simulink model "Architecture"  (R2025b)
settings: configuration reference "simulation" (kept outside this file)
StopFcn:
  | sim("models\PlaybackMechExplorer");
settings Model: DataDictionary=test.sldd  Creator=rpumpo  LastModifiedBy=rpumpo
settings ConfigSetRef: SourceName=simulation

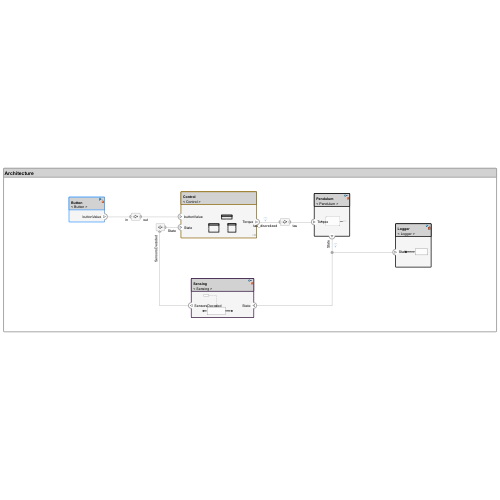
[thumbnail: Simulink's stored preview of the top-level diagram]
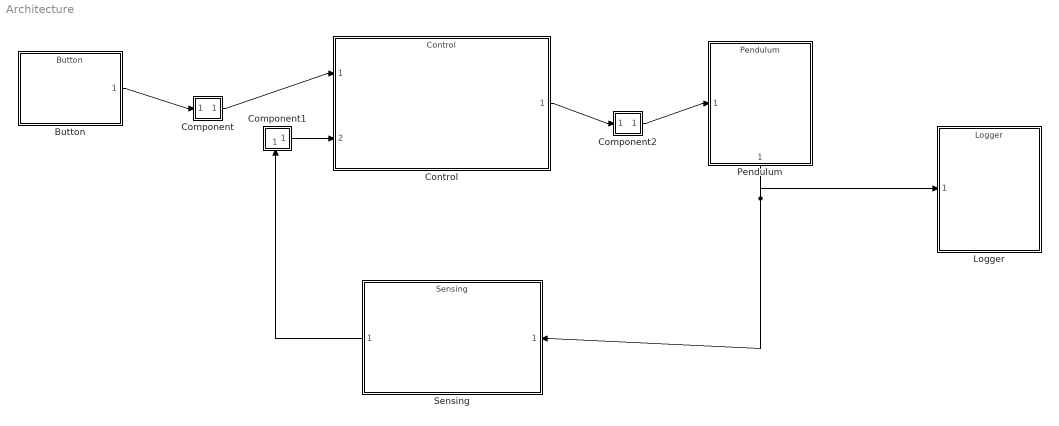
== system Architecture ==
  Button : ModelReference  ModelNameDialog=Button  SimulationMode=Normal  ModelReferenceVersion=1.6
      settings: PortSchema="{\"entries\":[{\"content\":{\"headerSize\":38,\"margin\":15,\"minimumSpacing\":25,\"sides\":[{\"content\":{},\"type\":\"ConnectorPlacement.EquallySpacedRectSide\",\"uuid\":\"8ec1d587-685a-426d-afd8-122ee0061f4c\"},{\"content\":{\"connectorIds\":[\"Out1\"],\"side\":\"RIGHT\"},\"type\":\"ConnectorPlacement.EquallySpacedRectSide\",\"uuid\":\"676e5b40-739e-4f92-aeaf-bee5408ade44\"},{\"content\":{\"side\":\"TOP\"},\"type\":\"ConnectorPlacement.EquallySpacedRectSide\",\"uuid\":\"01bc015e-a21d-4ad7-afeb-e19c798ece57\"}]},\"type\":\"ConnectorPlacement.EquallySpacedConnector\",\"uuid\":\"c5b56a8a-bb96-4a1a-b5ae-768463cc4daa\"}],\"packageUris\":[\"http://schema.mathworks.com/mf0/Connector/R2020b\"],\"version\":\"1.0\"}"
  Component : Subsystem
      settings: PortSchema="{\"entries\":[{\"content\":{\"margin\":10,\"minimumSpacing\":15,\"sides\":[{\"content\":{\"connectorIds\":[\"In1\"]},\"type\":\"ConnectorPlacement.EquallySpacedRectSide\",\"uuid\":\"52fbcab2-77e6-4c43-8240-cdc79aed3b18\"},{\"content\":{\"connectorIds\":[\"Out1\"],\"side\":\"RIGHT\"},\"type\":\"ConnectorPlacement.EquallySpacedRectSide\",\"uuid\":\"cdca0b56-8fb5-4ee8-9ac9-94cbfddd1752\"},{\"content\":{\"side\":\"TOP\"},\"type\":\"ConnectorPlacement.EquallySpacedRectSide\",\"uuid\":\"eb715b44-d91d-4d1d-af0d-8b01d7a8babe\"}]},\"type\":\"ConnectorPlacement.EquallySpacedConnector\",\"uuid\":\"fecc88ef-e61f-4ca4-bc17-41110eeb9f29\"}],\"packageUris\":[\"http://schema.mathworks.com/mf0/Connector/R2020b\"],\"version\":\"1.0\"}"
  Component1 : Subsystem
      settings: PortSchema="{\"entries\":[{\"content\":{\"margin\":10,\"minimumSpacing\":15,\"sides\":[{\"content\":{},\"type\":\"ConnectorPlacement.EquallySpacedRectSide\",\"uuid\":\"52fbcab2-77e6-4c43-8240-cdc79aed3b18\"},{\"content\":{\"connectorIds\":[\"Out1\"],\"side\":\"RIGHT\"},\"type\":\"ConnectorPlacement.EquallySpacedRectSide\",\"uuid\":\"cdca0b56-8fb5-4ee8-9ac9-94cbfddd1752\"},{\"content\":{\"side\":\"TOP\"},\"type\":\"ConnectorPlacement.EquallySpacedRectSide\",\"uuid\":\"eb715b44-d91d-4d1d-af0d-8b01d7a8babe\"},{\"content\":{\"connectorIds\":[\"In1\"],\"side\":\"BOTTOM\"},\"type\":\"ConnectorPlacement.EquallySpacedRectSide\",\"uuid\":\"c2091c5b-8a67-42b6-aad5-651c68393b83\"}]},\"type\":\"ConnectorPlacement.EquallySpacedConnector\",\"uuid\":\"fecc88ef-e61f-4ca4-bc17-41110eeb9f29\"}],\"packageUris\":[\"http://schema.mathworks.com/mf0/Connector/R2020b\"],\"version\":\"1.0\"}"
  Component2 : Subsystem
      settings: PortSchema="{\"entries\":[{\"content\":{\"margin\":10,\"minimumSpacing\":15,\"sides\":[{\"content\":{\"connectorIds\":[\"In1\"]},\"type\":\"ConnectorPlacement.EquallySpacedRectSide\",\"uuid\":\"52fbcab2-77e6-4c43-8240-cdc79aed3b18\"},{\"content\":{\"connectorIds\":[\"Out1\"],\"side\":\"RIGHT\"},\"type\":\"ConnectorPlacement.EquallySpacedRectSide\",\"uuid\":\"cdca0b56-8fb5-4ee8-9ac9-94cbfddd1752\"},{\"content\":{\"side\":\"TOP\"},\"type\":\"ConnectorPlacement.EquallySpacedRectSide\",\"uuid\":\"eb715b44-d91d-4d1d-af0d-8b01d7a8babe\"}]},\"type\":\"ConnectorPlacement.EquallySpacedConnector\",\"uuid\":\"fecc88ef-e61f-4ca4-bc17-41110eeb9f29\"}],\"packageUris\":[\"http://schema.mathworks.com/mf0/Connector/R2020b\"],\"version\":\"1.0\"}"
  Control : ModelReference  ModelNameDialog=Control  SimulationMode=Normal  ScheduleRates=on  ModelReferenceVersion=1.56
      settings: PortSchema="{\"entries\":[{\"content\":{\"headerSize\":38,\"margin\":15,\"minimumSpacing\":25,\"sides\":[{\"content\":{\"connectorIds\":[\"In1\",\"In2\"]},\"type\":\"ConnectorPlacement.EquallySpacedRectSide\",\"uuid\":\"863a0b16-e36b-44d6-9477-1468a80c696d\"},{\"content\":{\"connectorIds\":[\"Out1\"],\"side\":\"RIGHT\"},\"type\":\"ConnectorPlacement.EquallySpacedRectSide\",\"uuid\":\"ac9067ee-3fe6-46b1-b4d3-b466d54413ae\"},{\"content\":{\"side\":\"TOP\"},\"type\":\"ConnectorPlacement.EquallySpacedRectSide\",\"uuid\":\"d4aa2d7a-4362-47d2-9788-fc41168b683c\"}]},\"type\":\"ConnectorPlacement.EquallySpacedConnector\",\"uuid\":\"884a1123-87f2-4a92-8ca9-5d4169531818\"}],\"packageUris\":[\"http://schema.mathworks.com/mf0/Connector/R2020b\"],\"version\":\"1.0\"}"
  Logger : ModelReference  ModelNameDialog=Logger.slx  SimulationMode=Normal  ModelReferenceVersion=1.9
      settings: PortSchema="{\"entries\":[{\"content\":{\"headerSize\":38,\"margin\":15,\"minimumSpacing\":25,\"sides\":[{\"content\":{\"connectorIds\":[\"In1\"]},\"type\":\"ConnectorPlacement.EquallySpacedRectSide\",\"uuid\":\"e3850213-7836-4a76-9138-db9561f2dfa3\"},{\"content\":{\"side\":\"RIGHT\"},\"type\":\"ConnectorPlacement.EquallySpacedRectSide\",\"uuid\":\"0376d83e-b2c6-47e1-ac72-ef48c291ef7a\"},{\"content\":{\"side\":\"TOP\"},\"type\":\"ConnectorPlacement.EquallySpacedRectSide\",\"uuid\":\"0ca152af-581b-44cc-8c1a-1940fec58944\"},{\"content\":{\"side\":\"BOTTOM\"},\"type\":\"ConnectorPlacement.EquallySpacedRectSide\",\"uuid\":\"58a901f2-a9fb-4ea5-a869-3facdef2b65b\"}]},\"type\":\"ConnectorPlacement.EquallySpacedConnector\",\"uuid\":\"7f3a45e2-30ac-43d0-98f3-5299d75cc4ed\"}],\"packageUris\":[\"http://schema.mathworks.com/mf0/Connector/R2020b\"],\"version\":\"1.0\"}"
  Pendulum : ModelReference  ModelNameDialog=Pendulum  SimulationMode=Normal  ModelReferenceVersion=1.26
      settings: PortSchema="{\"entries\":[{\"content\":{\"headerSize\":38,\"margin\":15,\"minimumSpacing\":25,\"sides\":[{\"content\":{\"connectorIds\":[\"In1\"]},\"type\":\"ConnectorPlacement.EquallySpacedRectSide\",\"uuid\":\"de57860b-0736-4135-a3e8-86dccc8271d5\"},{\"content\":{\"side\":\"RIGHT\"},\"type\":\"ConnectorPlacement.EquallySpacedRectSide\",\"uuid\":\"36ab646b-84bc-41af-8fac-a30bd324c6d3\"},{\"content\":{\"side\":\"TOP\"},\"type\":\"ConnectorPlacement.EquallySpacedRectSide\",\"uuid\":\"400916d0-a027-46ef-830f-ede2528573e4\"},{\"content\":{\"connectorIds\":[\"Out1\"],\"side\":\"BOTTOM\"},\"type\":\"ConnectorPlacement.EquallySpacedRectSide\",\"uuid\":\"00a68dd3-bf65-408f-b5a8-975bdf578244\"}]},\"type\":\"ConnectorPlacement.EquallySpacedConnector\",\"uuid\":\"8bf5b967-d017-4010-a731-66d331b6151a\"}],\"packageUris\":[\"http://schema.mathworks.com/mf0/Connector/R2020b\"],\"version\":\"1.0\"}"
  Sensing : ModelReference  ModelNameDialog=Sensing  SimulationMode=Normal  ScheduleRates=on  CachedPortDiscreteRates=[-1]  ModelReferenceVersion=1.10
      settings: PortSchema="{\"entries\":[{\"content\":{\"headerSize\":38,\"margin\":15,\"minimumSpacing\":25,\"sides\":[{\"content\":{\"connectorIds\":[\"Out1\"]},\"type\":\"ConnectorPlacement.EquallySpacedRectSide\",\"uuid\":\"863a0b16-e36b-44d6-9477-1468a80c696d\"},{\"content\":{\"connectorIds\":[\"In1\"],\"side\":\"RIGHT\"},\"type\":\"ConnectorPlacement.EquallySpacedRectSide\",\"uuid\":\"ac9067ee-3fe6-46b1-b4d3-b466d54413ae\"},{\"content\":{\"side\":\"TOP\"},\"type\":\"ConnectorPlacement.EquallySpacedRectSide\",\"uuid\":\"d4aa2d7a-4362-47d2-9788-fc41168b683c\"},{\"content\":{\"side\":\"HIDDEN\"},\"type\":\"ConnectorPlacement.EquallySpacedRectSide\",\"uuid\":\"a4bb201e-c22d-4356-a85f-9b291461f392\"}]},\"type\":\"ConnectorPlacement.EquallySpacedConnector\",\"uuid\":\"884a1123-87f2-4a92-8ca9-5d4169531818\"}],\"packageUris\":[\"http://schema.mathworks.com/mf0/Connector/R2020b\"],\"version\":\"1.0\"}"
  wires:
  Sensing/1 -> Component1/1(SensorsDecoded)
  Component1/1(State) -> Control/2
  Control/1 -> Component2/1(tau_discretized)
  Component2/1(tau) -> Pendulum/1
  Component/1(out) -> Control/1
  Button/1 -> Component/1(in)
  Pendulum/1 -> Sensing/1, Logger/1

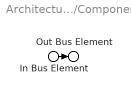
== system Architecture/Component ==
  In Bus Element : Inport  PortName=in
  Out Bus Element : Outport  PortName=out
  wires:
  In Bus Element/1 -> Out Bus Element/1

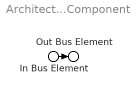
== system Architecture/Component1 ==
  In Bus Element : Inport  PortName=SensorsDecoded
  Out Bus Element : Outport  PortName=State
  wires:
  In Bus Element/1 -> Out Bus Element/1

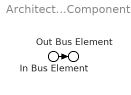
== system Architecture/Component2 ==
  In Bus Element : Inport  PortName=tau_discretized
  Out Bus Element : Outport  PortName=tau
  wires:
  In Bus Element/1 -> Out Bus Element/1
